simulink model "problem7"  (R2020b)
settings: Solver=VariableStepAuto  StartTime=0.0  StopTime=10.0  RelTol=1e-3
settings Model: Creator=Shree  LastModifiedBy=Shree

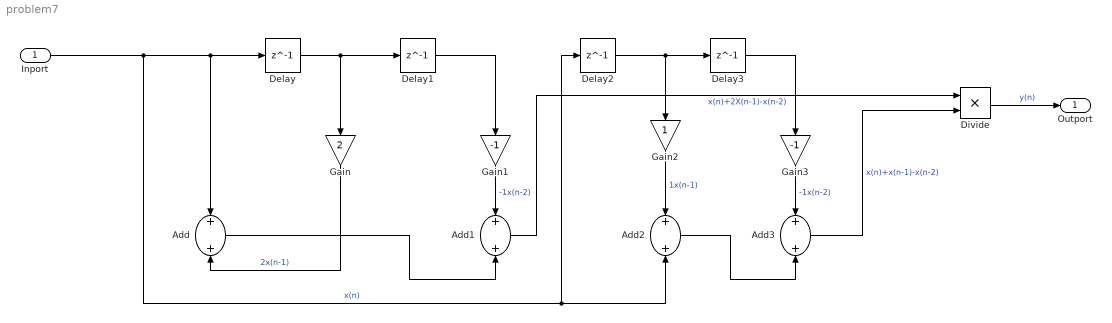
== system problem7 ==
  Inport : Inport
  Add{,1..3} (4 alike) : Sum
  Delay{,1..3} (4 alike) : Delay  DelayLength=1
  Divide : Product  Inputs=**
  Gain : Gain  Gain=2
  Gain1 : Gain  Gain=-1
  Gain2 : Gain
  Gain3 : Gain  Gain=-1
  Outport : Outport
  wires:
  Inport/1 -> Delay2/1, Add2/2, Add/1, Delay/1  "x(n)"
  Delay/1 -> Gain/1, Delay1/1
  Delay1/1 -> Gain1/1
  Gain1/1 -> Add1/1  "-1x(n-2)"
  Gain/1 -> Add/2  "2x(n-1)"
  Add/1 -> Add1/2
  Delay2/1 -> Gain2/1, Delay3/1
  Gain2/1 -> Add2/1  "1x(n-1)"
  Add2/1 -> Add3/2
  Delay3/1 -> Gain3/1
  Gain3/1 -> Add3/1  "-1x(n-2)"
  Divide/1 -> Outport/1  "y(n)"
  Add3/1 -> Divide/2  "x(n)+x(n-1)-x(n-2)"
  Add1/1 -> Divide/1  "x(n)+2X(n-1)-x(n-2)"
